simulink model "Regler_Kaskadierung"  (R2017b)
settings: Solver=FixedStepAuto  StartTime=0.0  StopTime=24000  FixedStep=0.5  RelTol=1e-3
values from neighbouring files (symbols this model uses):
  Kd_Z = Zelle.Kd    [Regler_Kaskadierung.m]
  Ki_M = Kp_M/Tn_M    (= 1.47286821705)    [Regler_Kaskadierung.m]    (also in Regler_Mantel.m = Kp_M/Tn_M)
  Ki_Z = Zelle.Ki    [Regler_Kaskadierung.m]
  Kp_M = (0.35/K_Mantel)*(T1_Mantel/Tu)    (= 1.76744186047)    [Regler_Kaskadierung.m]    (also in Regler_Kaskadierung_2.m = 5; Regler_Kaskadierung_2_editor.m = 5; Regler_Mantel.m = (0.35/K_Mantel)*(T1_Mantel/Tu))
  Kp_Z = Zelle.Kp    [Regler_Kaskadierung.m]
  Tn_M = 1.2*Tu    (= 1.2)    [Regler_Kaskadierung.m]    (also in Regler_Mantel.m = 1.2*Tu)
  Tt_Z = sqrt(Tn_Z*Tv_Z)    [Regler_Kaskadierung.m]
libraries: cstblocks x2, simulink x1
settings Model: Creator=arbno  LastModifiedBy=arbno

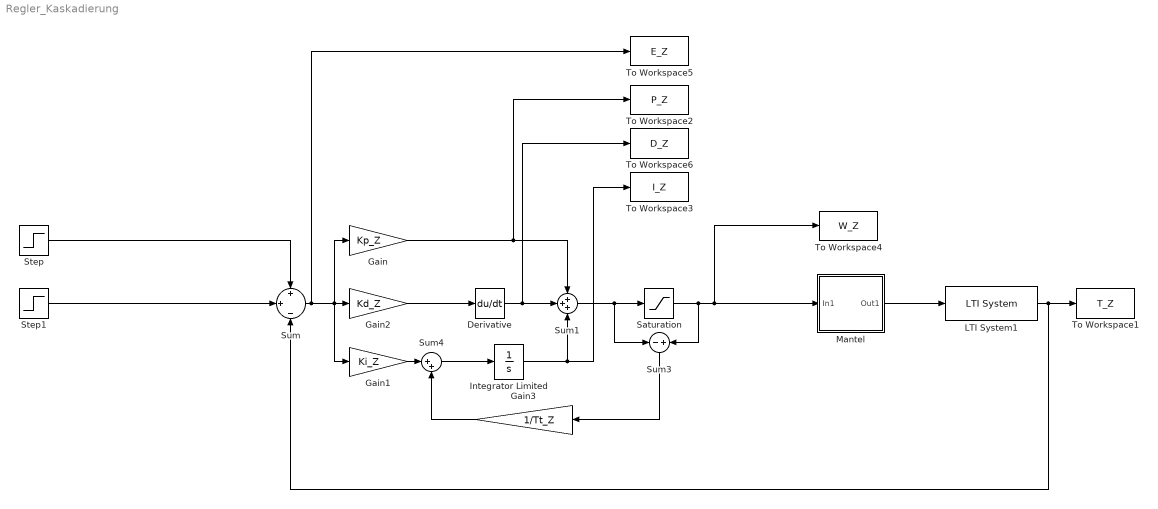
== system Regler_Kaskadierung ==
  Derivative : Derivative
  Gain : Gain  Gain=Kp_Z
  Gain1 : Gain  Gain=Ki_Z
  Gain2 : Gain  Gain=Kd_Z
  Gain3 : Gain  Gain=1/Tt_Z
  Integrator Limited : Integrator  UpperSaturationLimit=150  LowerSaturationLimit=-150
  LTI System1 : cstblocks/LTI System  sys=G_Zelle  IC=[]
  Mantel : Subsystem
  Saturation : Saturate  UpperLimit=141  LowerLimit=0
  Step : Step  Time=0  After=80  SampleTime=0
  Step1 : Step  Time=0  After=0  SampleTime=0
  Sum : Sum  Inputs=+|+|-
  Sum1 : Sum  Inputs=+++
  Sum3 : Sum  Inputs=-|+
  Sum4 : Sum  Inputs=|++
  To Workspace1 : ToWorkspace  VariableName=T_Z  SaveFormat=Structure With Time  SampleTime=-1
  To Workspace2 : ToWorkspace  VariableName=P_Z  SaveFormat=Structure With Time  SampleTime=-1
  To Workspace3 : ToWorkspace  VariableName=I_Z  SaveFormat=Structure With Time  SampleTime=-1
  To Workspace4 : ToWorkspace  VariableName=W_Z  SaveFormat=Structure With Time  SampleTime=-1
  To Workspace5 : ToWorkspace  VariableName=E_Z  SaveFormat=Structure With Time  SampleTime=-1
  To Workspace6 : ToWorkspace  VariableName=D_Z  SaveFormat=Structure With Time  SampleTime=-1
  wires:
  Mantel/1(Out1) -> LTI System1/1
  Gain2/1 -> Derivative/1
  LTI System1/1 -> To Workspace1/1, Sum/3
  Sum1/1 -> Sum3/1, Saturation/1
  Step/1 -> Sum/1
  Derivative/1 -> To Workspace6/1, Sum1/2
  Sum4/1 -> Integrator Limited/1
  Sum/1 -> To Workspace5/1, Gain1/1, Gain2/1, Gain/1
  Gain/1 -> Sum1/1, To Workspace2/1
  Saturation/1 -> Sum3/2, Mantel/1(In1), To Workspace4/1
  Integrator Limited/1 -> To Workspace3/1, Sum1/3
  Sum3/1 -> Gain3/1
  Gain1/1 -> Sum4/1
  Gain3/1 -> Sum4/2
  Step1/1 -> Sum/2

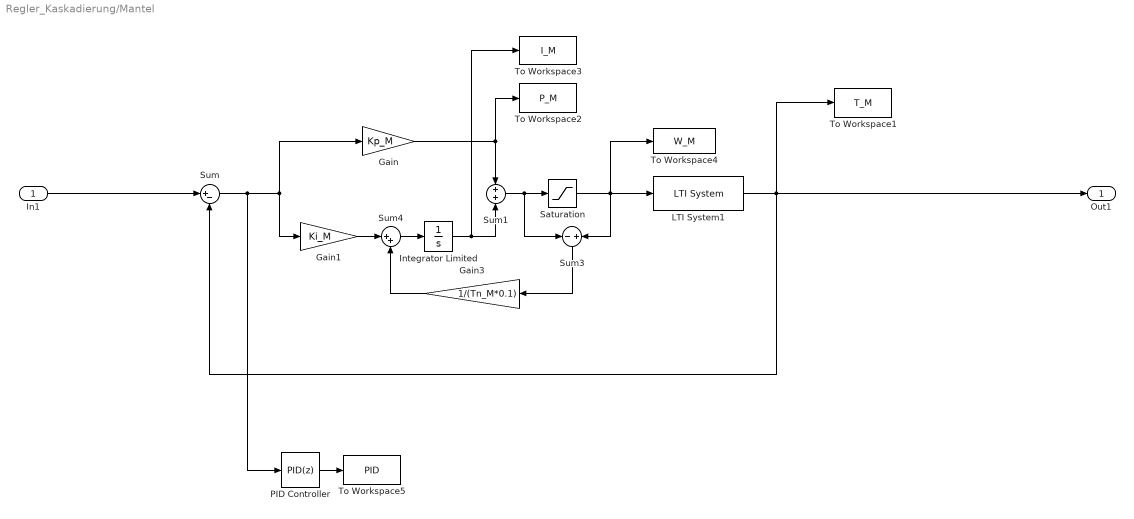
== system Regler_Kaskadierung/Mantel ==
  In1 : Inport
  Gain : Gain  Gain=Kp_M
  Gain1 : Gain  Gain=Ki_M
  Gain3 : Gain  Gain=1/(Tn_M*0.1)
  Integrator Limited : Integrator  UpperSaturationLimit=0.5  LowerSaturationLimit=-0.5
  LTI System1 : cstblocks/LTI System  sys=G_Mantel  IC=[]
  PID Controller : simulink/Continuous/PID Controller  Controller=PID  TimeDomain=Discrete-time  SampleTime=-1  IntegratorMethod=Forward Euler  FilterMethod=Forward Euler  Form=Parallel  UseFilter=on  ControllerParametersSource=internal  P=Kp_M  I=Ki_M  D=0  N=100  InitialConditionSource=internal  InitialConditionForIntegrator=0  InitialConditionForFilter=0  ExternalReset=none  LimitOutput=on  UpperSaturationLimit=11000  LowerSaturationLimit=0  LinearizeAsGain=off  AntiWindupMode=clamping  Kb=1  TrackingMode=off  Kt=1  PParamMin=[]  PParamMax=[]  IParamMin=[]  IParamMax=[]  DParamMin=[]  DParamMax=[]  NParamMin=[]  NParamMax=[]  KbParamMin=[]  KbParamMax=[]  KtParamMin=[]  KtParamMax=[]  POutMin=[]  POutMax=[]  IOutMin=[]  IOutMax=[]  DOutMin=[]  DOutMax=[]  NOutMin=[]  NOutMax=[]  KbOutMin=[]  KbOutMax=[]  KtOutMin=[]  KtOutMax=[]  IntegratorOutMin=[]  IntegratorOutMax=[]  FilterOutMin=[]  FilterOutMax=[]  SumOutMin=[]  SumOutMax=[]  SumI1OutMin=[]  SumI1OutMax=[]  SumI2OutMin=[]  SumI2OutMax=[]  SumI3OutMin=[]  SumI3OutMax=[]  SumDOutMin=[]  SumDOutMax=[]  SaturationOutMin=[]  SaturationOutMax=[]  IntegratorContinuousStateAttributes=''  IntegratorStateMustResolveToSignalObject=off  IntegratorRTWStateStorageClass=Auto  FilterContinuousStateAttributes=''  FilterStateMustResolveToSignalObject=off  FilterRTWStateStorageClass=Auto  DifferentiatorICPrevScaledInput=0  DifferentiatorOutMin=[]  DifferentiatorOutMax=[]  InitialConditionSetting=State (most efficient)  FilterDiffOutCoefMin=[]  FilterDiffOutCoefMax=[]  SumDenOutMin=[]  SumDenOutMax=[]  SumNumOutMin=[]  SumNumOutMax=[]  ReciprocalOutMin=[]  ReciprocalOutMax=[]  DivideOutMin=[]  DivideOutMax=[]  TunerSelectOption=Frequency Response Based
  Saturation : Saturate  UpperLimit=1  LowerLimit=0
  Sum : Sum  Inputs=|+-
  Sum1 : Sum
  Sum3 : Sum  Inputs=-|+
  Sum4 : Sum  Inputs=|++
  To Workspace1 : ToWorkspace  VariableName=T_M  SaveFormat=Structure With Time  SampleTime=-1
  To Workspace2 : ToWorkspace  VariableName=P_M  SaveFormat=Structure With Time  SampleTime=-1
  To Workspace3 : ToWorkspace  VariableName=I_M  SaveFormat=Structure With Time  SampleTime=-1
  To Workspace4 : ToWorkspace  VariableName=W_M  SaveFormat=Structure With Time  SampleTime=-1
  To Workspace5 : ToWorkspace  VariableName=PID  SaveFormat=Structure With Time  SampleTime=-1
  Out1 : Outport
  wires:
  LTI System1/1 -> Out1/1, Sum/2, To Workspace1/1
  Integrator Limited/1 -> To Workspace3/1, Sum1/2
  Sum/1 -> Gain/1, Gain1/1, PID Controller/1
  In1/1 -> Sum/1
  PID Controller/1 -> To Workspace5/1
  Gain/1 -> Sum1/1, To Workspace2/1
  Gain3/1 -> Sum4/2
  Saturation/1 -> LTI System1/1, Sum3/2, To Workspace4/1
  Sum1/1 -> Sum3/1, Saturation/1
  Sum3/1 -> Gain3/1
  Gain1/1 -> Sum4/1
  Sum4/1 -> Integrator Limited/1
